simulink model "lindiscrmodel_val"  (R2019a)
settings: Solver=VariableStepAuto  StartTime=0.0  StopTime=30  RelTol=1e-3
InitFcn:
  | lin_discr_model
values from neighbouring files (symbols this model uses):
  Ts = 0.01    [lindiscrmodel.m]
  xref = B_eq1_d_val(:,3)    [lindiscrmodel.m]
undefined symbols (not defined in the file or in its folder): A_eq1_d_val, B_eq1_d2_val, C_eq1_d_val, L_val
settings Model: Creator=jessi  LastModifiedBy=jessi

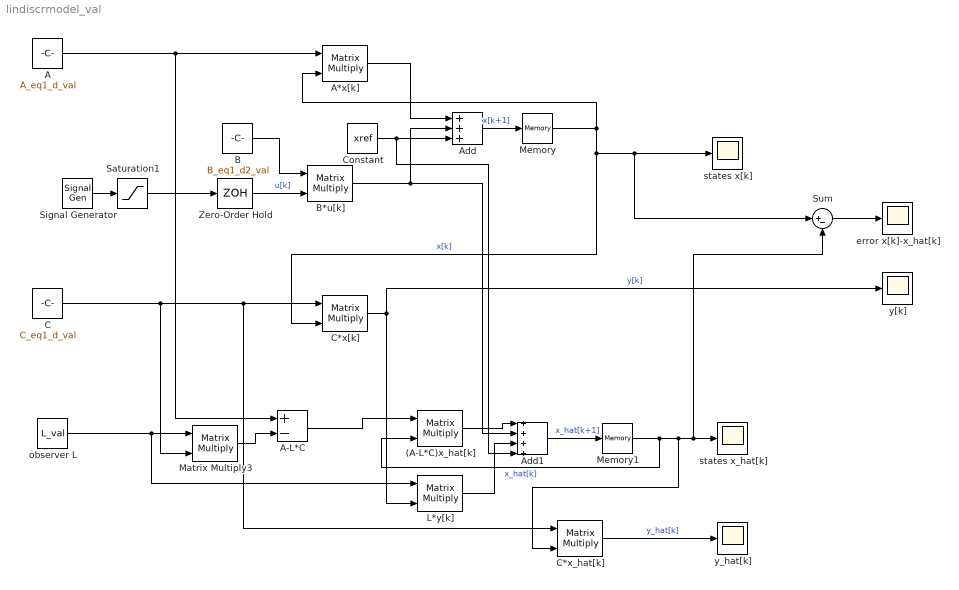
== system lindiscrmodel_val ==
  (A-L*C)x_hat[k] : Product  Multiplication=Matrix(*)
  A : Constant  Value=A_eq1_d_val  SampleTime=Ts
  A*x[k] : Product  Multiplication=Matrix(*)
  A-L*C : Sum  Inputs=+-
  Add : Sum  Inputs=+++
  Add1 : Sum  Inputs=++++
  B : Constant  Value=B_eq1_d2_val  SampleTime=Ts
  B*u[k] : Product  Multiplication=Matrix(*)
  C : Constant  Value=C_eq1_d_val  SampleTime=Ts
  C*x[k] : Product  Multiplication=Matrix(*)
  C*x_hat[k] : Product  Multiplication=Matrix(*)
  Constant : Constant  Value=xref  SampleTime=Ts
  L*y[k] : Product  Multiplication=Matrix(*)
  Matrix Multiply3 : Product  Multiplication=Matrix(*)
  Memory : Memory  InitialCondition=[pi;0;0;0]
  Memory1 : Memory  InitialCondition=[pi;0;0;0]
  Saturation1 : Saturate  UpperLimit=1  LowerLimit=-1
  Signal Generator : SignalGenerator  WaveForm=square  Amplitude=-0.3
  Sum : Sum  Inputs=|+-
  Zero-Order Hold : ZeroOrderHold  SampleTime=Ts
  error x[k]-x_hat[k] : Scope
  observer L : Constant  Value=L_val  SampleTime=Ts
  states x[k] : Scope
  states x_hat[k] : Scope
  y[k] : Scope
  y_hat[k] : Scope
  wires:
  Signal Generator/1 -> Saturation1/1
  Zero-Order Hold/1 -> B*u[k]/2  "u[k]"
  B/1 -> B*u[k]/1
  A/1 -> A-L*C/1, A*x[k]/1
  A*x[k]/1 -> Add/1
  B*u[k]/1 -> Add1/2, Add/2
  Memory/1 -> A*x[k]/2, Sum/1, states x[k]/1, C*x[k]/2  "x[k]"
  C/1 -> Matrix Multiply3/2, C*x_hat[k]/1, C*x[k]/1
  C*x[k]/1 -> L*y[k]/2, y[k]/1  "y[k]"
  observer L/1 -> L*y[k]/1, Matrix Multiply3/1
  Matrix Multiply3/1 -> A-L*C/2
  A-L*C/1 -> (A-L*C)x_hat[k]/1
  (A-L*C)x_hat[k]/1 -> Add1/1
  L*y[k]/1 -> Add1/3
  Add1/1 -> Memory1/1  "x_hat[k+1]"
  Memory1/1 -> C*x_hat[k]/2, Sum/2, states x_hat[k]/1, (A-L*C)x_hat[k]/2  "x_hat[k]"
  C*x_hat[k]/1 -> y_hat[k]/1  "y_hat[k]"
  Saturation1/1 -> Zero-Order Hold/1
  Add/1 -> Memory/1  "x[k+1]"
  Constant/1 -> Add1/4, Add/3
  Sum/1 -> error x[k]-x_hat[k]/1
